simulink model "dkPID"  (Simulink 7.4)
settings: Solver=ode45  StartTime=0.0  StopTime=600  RelTol=1e-3
settings Model: Creator=phuck  LastModifiedBy=phuck

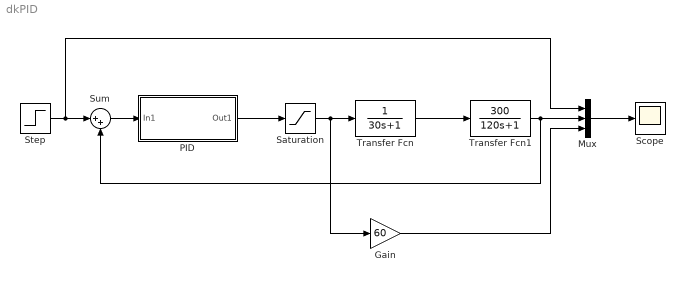
== system dkPID ==
  Gain : Gain  Gain=60  ParameterDataType=fixdt(1, 16)  ParameterScaling=2^0  OutDataType=fixdt(1, 16)  OutScaling=2^0
  Mux : Mux  Inputs=3
  PID : Subsystem
  Saturation : Saturate  OutDataType=fixdt(1, 16)  OutScaling=2^0
  Scope : Scope
  Step : Step  Time=0  After=100  SampleTime=0
  Sum : Sum  Inputs=|++  OutDataType=fixdt(1, 16)  OutScaling=2^0
  Transfer Fcn : TransferFcn  Denominator=[30 1]
  Transfer Fcn1 : TransferFcn  Numerator=[300]  Denominator=[120 1]
  wires:
  Step/1 -> Sum/1, Mux/1
  Sum/1 -> PID/1(In1)
  PID/1(Out1) -> Saturation/1
  Saturation/1 -> Transfer Fcn/1, Gain/1
  Transfer Fcn/1 -> Transfer Fcn1/1
  Transfer Fcn1/1 -> Mux/2, Sum/2
  Mux/1 -> Scope/1
  Gain/1 -> Mux/3

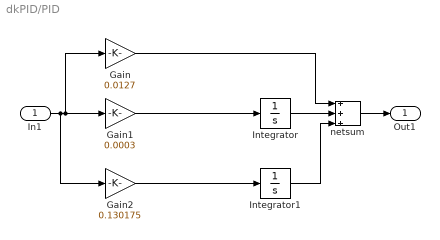
== system dkPID/PID ==
  In1 : Inport  OutDataType=fixdt(1, 16)  OutScaling=2^0
  Gain : Gain  Gain=0.0127  ParameterDataType=fixdt(1, 16)  ParameterScaling=2^0  OutDataType=fixdt(1, 16)  OutScaling=2^0
  Gain1 : Gain  Gain=0.0003  ParameterDataType=fixdt(1, 16)  ParameterScaling=2^0  OutDataType=fixdt(1, 16)  OutScaling=2^0
  Gain2 : Gain  Gain=0.130175  ParameterDataType=fixdt(1, 16)  ParameterScaling=2^0  OutDataType=fixdt(1, 16)  OutScaling=2^0
  Integrator : Integrator
  Integrator1 : Integrator
  netsum : Sum  Inputs=3  OutDataType=sfix(16)  OutScaling=2^0  SaturateOnIntegerOverflow=on  InputSameDT=on  OutDataTypeStr=Inherit: Same as first input
  Out1 : Outport  OutDataType=fixdt(1, 16)  OutScaling=2^0
  wires:
  In1/1 -> Gain1/1, Gain/1, Gain2/1
  Gain/1 -> netsum/1
  Gain1/1 -> Integrator/1
  Integrator/1 -> netsum/2
  netsum/1 -> Out1/1
  Integrator1/1 -> netsum/3
  Gain2/1 -> Integrator1/1
